simulink model "Force_control_impedance"  (R2020b)
settings: Solver=VariableStepAuto  StartTime=0.0  StopTime=.1  RelTol=1e-3
settings Model: Creator=Jae  LastModifiedBy=Jae

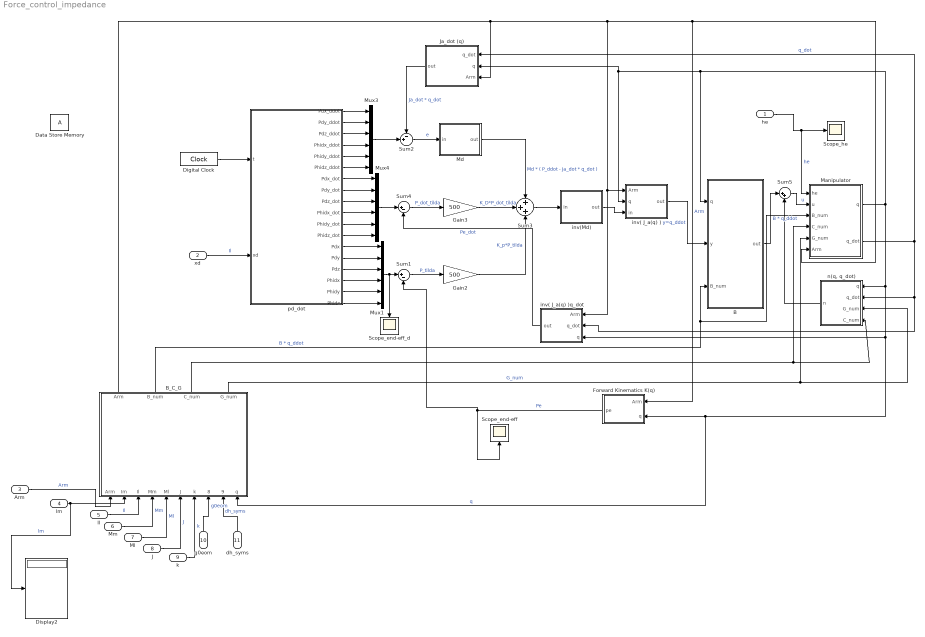
== system Force_control_impedance ==
  he : Inport  PortDimensions=6  SampleTime=0.01
  xd : Inport  Port=2  PortDimensions=6  SampleTime=0.01
  Arm : Inport  Port=3  PortDimensions=6  SampleTime=0.01
  lm : Inport  Port=4  PortDimensions=6  SampleTime=0.01
  Il : Inport  Port=5  PortDimensions=6  SampleTime=0.01
  Mm : Inport  Port=6  PortDimensions=6  SampleTime=0.01
  Ml : Inport  Port=7  PortDimensions=6  SampleTime=0.01
  J : Inport  Port=8  PortDimensions=6  SampleTime=0.01
  k : Inport  Port=9  PortDimensions=6  SampleTime=0.01
  g0eom : Inport  Port=10  PortDimensions=6  SampleTime=0.01
  dh_syms : Inport  Port=11  PortDimensions=6  SampleTime=0.01
  B : MATLAB Function  TreatAsAtomicUnit=on
  B_C_G : MATLAB Function  TreatAsAtomicUnit=on
  Data Store Memory : DataStoreMemory  ReadBeforeWriteMsg=warning  WriteAfterWriteMsg=warning  WriteAfterReadMsg=warning  ShowAdditionalParam=off
  Digital Clock : DigitalClock  SampleTime=0.01
  Display2 : Display
  Forward Kinematics K(q) : MATLAB Function  TreatAsAtomicUnit=on
  Gain2 : Gain  Gain=500
  Gain3 : Gain  Gain=500
  Ja_dot (q) : MATLAB Function  TreatAsAtomicUnit=on
  Manipulator : Subsystem
  Md : MATLAB Function  TreatAsAtomicUnit=on
  Mux1 : Mux  Inputs=6
  Mux3 : Mux  Inputs=6
  Mux4 : Mux  Inputs=6
  Scope_end-eff : Scope
  Scope_end-eff_d : Scope
  Scope_he : Scope
  Sum1 : Sum  Inputs=|+-
  Sum2 : Sum  Inputs=-+|
  Sum3 : Sum  Inputs=+++
  Sum4 : Sum  Inputs=|+-
  Sum5 : Sum  Inputs=|++
  inv( J_a(q) ) : MATLAB Function  TreatAsAtomicUnit=on
  inv( J_a(q) )q_dot : MATLAB Function  TreatAsAtomicUnit=on
  inv(Md) : MATLAB Function  TreatAsAtomicUnit=on
  "n(q, q_dot)" : Subsystem
  pd_dot : MATLAB Function  TreatAsAtomicUnit=on
  wires:
  Digital Clock/1 -> pd_dot/1(t)
  inv( J_a(q) )/1(out) -> B/2(y)  "y=q_ddot"
  pd_dot/13(Pdx) -> Mux1/1
  pd_dot/14(Pdy) -> Mux1/2
  pd_dot/15(Pdz) -> Mux1/3
  pd_dot/16(Phidx) -> Mux1/4
  pd_dot/17(Phidy) -> Mux1/5
  pd_dot/18(Phidz) -> Mux1/6
  pd_dot/1(Pdx_ddot) -> Mux3/1
  pd_dot/2(Pdy_ddot) -> Mux3/2
  pd_dot/3(Pdz_ddot) -> Mux3/3
  pd_dot/4(Phidx_ddot) -> Mux3/4
  pd_dot/5(Phidy_ddot) -> Mux3/5
  pd_dot/6(Phidz_ddot) -> Mux3/6
  pd_dot/7(Pdx_dot) -> Mux4/1
  pd_dot/8(Pdy_dot) -> Mux4/2
  pd_dot/9(Pdz_dot) -> Mux4/3
  pd_dot/10(Phidx_dot) -> Mux4/4
  pd_dot/11(Phidy_dot) -> Mux4/5
  pd_dot/12(Phidz_dot) -> Mux4/6
  Gain3/1 -> Sum3/2  "K_D*P_dot_tilda"
  Mux3/1 -> Sum2/2
  Sum2/1 -> Md/1(in)  "e"
  Md/1(out) -> Sum3/1  "Md * ( P_ddot - Ja_dot * q_dot )"
  Mux4/1 -> Sum4/1
  Sum4/1 -> Gain3/1  "P_dot_tilda"
  Mux1/1 -> Scope_end-eff_d/1, Sum1/1
  Sum1/1 -> Gain2/1  "P_tilda"
  Sum3/1 -> inv(Md)/1(in)
  Gain2/1 -> Sum3/3  "K_p*P_tilda"
  inv(Md)/1(out) -> inv( J_a(q) )/3(in)
  Ja_dot (q)/1(out) -> Sum2/1  "Ja_dot * q_dot"
  Forward Kinematics K(q)/1(pe) -> Sum1/2, Scope_end-eff/1  "Pe"
  inv( J_a(q) )q_dot/1(out) -> Sum4/2  "Pe_dot"
  B/1(out) -> Sum5/1  "B * q_ddot"
  "n(q, q_dot)"/1(n) -> Sum5/2
  Manipulator/1(q) -> B/1(q), inv( J_a(q) )/2(q), Ja_dot (q)/2(q), Forward Kinematics K(q)/2(q), B_C_G/10(q), inv( J_a(q) )q_dot/3(q), "n(q, q_dot)"/1(q)  "q"
  Manipulator/2(q_dot) -> Ja_dot (q)/1(q_dot), inv( J_a(q) )q_dot/2(q_dot), "n(q, q_dot)"/2(q_dot)  "q_dot"
  Sum5/1 -> Manipulator/2(u)  "u"
  he/1 -> Scope_he/1, Manipulator/1(he)  "he"
  Arm/1 -> B_C_G/1("Arm ")  "Arm"
  lm/1 -> Display2/1, B_C_G/2(Im)  "lm"
  Il/1 -> B_C_G/3(Il)  "Il"
  Mm/1 -> B_C_G/4(Mm)  "Mm"
  Ml/1 -> B_C_G/5(Ml)  "Ml"
  J/1 -> B_C_G/6(J)  "J"
  k/1 -> B_C_G/7(k)  "k"
  g0eom/1 -> B_C_G/8(g0eom)  "g0eom"
  dh_syms/1 -> B_C_G/9(dh_syms)  "dh_syms"
  B_C_G/2(B_num) -> B/3(B_num), Manipulator/3(B_num)  "B * q_ddot"
  B_C_G/1(Arm) -> Ja_dot (q)/3(Arm), Forward Kinematics K(q)/1(Arm), Manipulator/6(Arm), inv( J_a(q) )q_dot/1(Arm), inv( J_a(q) )/1(Arm)  "Arm"
  B_C_G/4(G_num) -> Manipulator/5(G_num), "n(q, q_dot)"/3(G_num)  "G_num"
  B_C_G/3(C_num) -> Manipulator/4(C_num), "n(q, q_dot)"/4(C_num)
  xd/1 -> pd_dot/2(xd)  "Il"

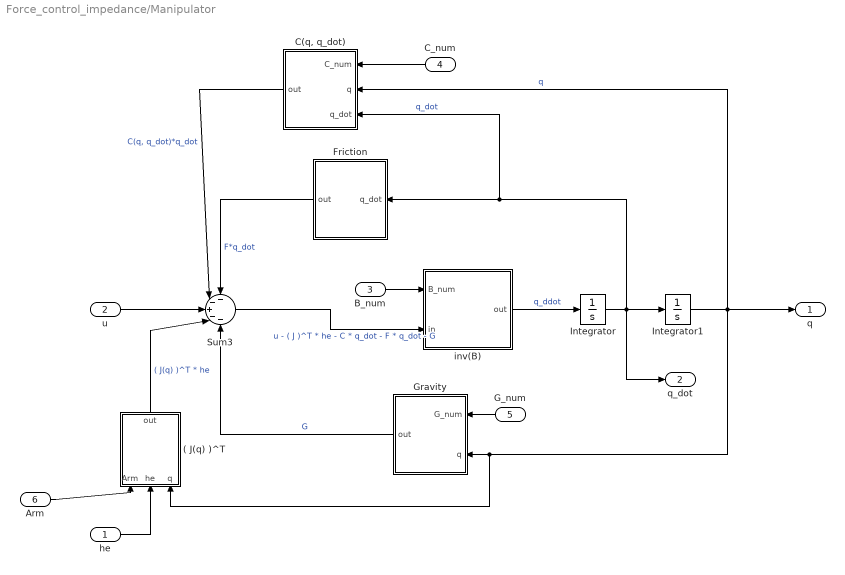
== system Force_control_impedance/Manipulator ==
  he : Inport
  u : Inport  Port=2
  B_num : Inport  Port=3
  C_num : Inport  Port=4
  G_num : Inport  Port=5
  Arm : Inport  Port=6
  ( J(q) )^T : MATLAB Function  TreatAsAtomicUnit=on
  "C(q, q_dot)" : MATLAB Function  TreatAsAtomicUnit=on
  Friction : MATLAB Function  TreatAsAtomicUnit=on
  Gravity : MATLAB Function  TreatAsAtomicUnit=on
  Integrator : Integrator  InitialCondition=[0 0 0 0 0 0]'  ZeroCross=off
  Integrator1 : Integrator  InitialCondition=[0 0 0 0 0 0]'  ZeroCross=off
  Sum3 : Sum  Inputs=--+--
  inv(B) : MATLAB Function  TreatAsAtomicUnit=on
  q : Outport
  q_dot : Outport  Port=2
  wires:
  u/1 -> Sum3/3
  ( J(q) )^T/1(out) -> Sum3/4  "( J(q) )^T * he"
  "C(q, q_dot)"/1(out) -> Sum3/2  "C(q, q_dot)*q_dot"
  Friction/1(out) -> Sum3/1  "F*q_dot"
  inv(B)/1(out) -> Integrator/1  "q_ddot"
  Integrator/1 -> Integrator1/1, q_dot/1, Friction/1(q_dot), "C(q, q_dot)"/3(q_dot)  "q_dot"
  Integrator1/1 -> Gravity/2(q), ( J(q) )^T/3(q), "C(q, q_dot)"/2(q), q/1  "q"
  Sum3/1 -> inv(B)/2(in)  "u - ( J )^T * he - C * q_dot - F * q_dot - G"
  Gravity/1(out) -> Sum3/5  "G"
  he/1 -> ( J(q) )^T/2(he)
  B_num/1 -> inv(B)/1(B_num)
  C_num/1 -> "C(q, q_dot)"/1(C_num)
  G_num/1 -> Gravity/1(G_num)
  Arm/1 -> ( J(q) )^T/1(Arm)

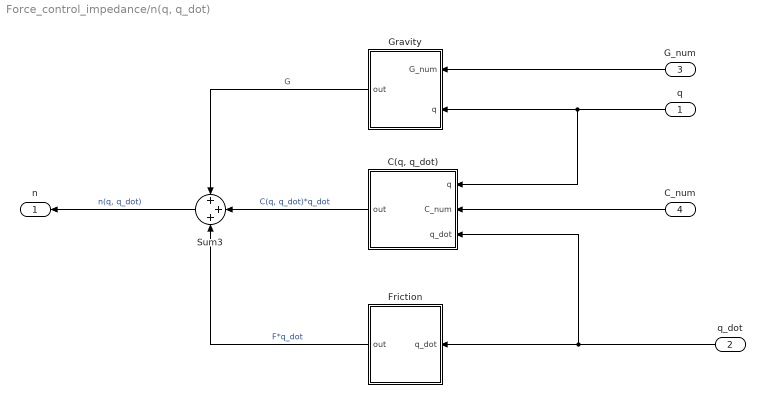
== system Force_control_impedance/n(q, q_dot) ==
  q : Inport
  q_dot : Inport  Port=2
  G_num : Inport  Port=3
  C_num : Inport  Port=4
  "C(q, q_dot)" : MATLAB Function  TreatAsAtomicUnit=on
  Friction : MATLAB Function  TreatAsAtomicUnit=on
  Gravity : MATLAB Function  TreatAsAtomicUnit=on
  Sum3 : Sum  Inputs=+++
  n : Outport
  wires:
  Sum3/1 -> n/1  "n(q, q_dot)"
  Gravity/1(out) -> Sum3/1  "G"
  "C(q, q_dot)"/1(out) -> Sum3/2  "C(q, q_dot)*q_dot"
  Friction/1(out) -> Sum3/3  "F*q_dot"
  q/1 -> "C(q, q_dot)"/1(q), Gravity/2(q)
  q_dot/1 -> "C(q, q_dot)"/3(q_dot), Friction/1(q_dot)
  G_num/1 -> Gravity/1(G_num)
  C_num/1 -> "C(q, q_dot)"/2(C_num)

== matlab function Force_control_impedance/inv( J_a(q) )q_dot ==
  data: Arm input; q_dot input; out output; q input
function out = Ja(Arm, q_dot, q)
%{
Inputs:
in: q_dot, q
    nx1    nx1             
Output: Ja*q_dot;
        6xn*nx1 = 6x1
%}
Ja = jacob0(Arm, q', 'rpy'); % 6xn

out = Ja*q_dot;
end

== matlab function Force_control_impedance/n(q, q_dot)/C(q, q_dot) ==
  data: q input; C_num input; q_dot input; out output
function out = C(q, C_num, q_dot)
% need to calculate C

out=C_num*q_dot;
end

== matlab function Force_control_impedance/n(q, q_dot)/Gravity ==
  data: G_num input; q input; out output
function out = G(G_num, q)
out=G_num;
end

== matlab function Force_control_impedance/n(q, q_dot)/Friction ==
  data: q_dot input; out output
function out = F(q_dot)
%{
Inputs:
in: q_dot
    nx1                
Output: F * q_dot;
        nxn*nx1 = nx1
%}
%NOTE: Assumed Arm,Im,Il,Mm,Ml,J,k,g0eom,dh_syms are global variables
%[B,C,G] = EOMFinder(Arm,Im,Il,Mm,Ml,J,k,g0eom,dh_syms);
%function Fv = Friction(FB, Fpos, Fneg, dq, n)
%F is friction is  NxN
%n=size(FB,1);
%assert (n <= 20);
%create vector of friction coefficients
n=length(q0)
FB=0; Fpos=0; Fneg=0; 
F_vector=zeros(n,1);

for i=1:n
    if dq(i)>0
        F_vector(i)= FB*dq(i)+Fpos;
    elseif dq(i)<0 % 
        F_vector(i)= FB*dq(i)+Fneg;
    else %         -        +
        F_vector(i)=0;
    end
end

%convert F_vector to diagonal matrix
F_diag=diag(F_vector);

%out is Nx1
out=zeros(n,1);
out=F_diag;

end

== matlab function Force_control_impedance/B_C_G ==
  data: Arm output; B_num output; Arm input; Im input; Il input; Mm input; Ml input; J input; k input; g0eom input; dh_syms input; q input; C_num output; G_num output
function [Arm, B_num, C_num, G_num] = B_C_G(Arm,Im,Il,Mm,Ml,J,k,g0eom,dh_syms, q)
%{
Inputs:
in: q,     y (q_ddot)
    nx1    nx1             
Output: B*y;
        nxn*nx1 = nx1
%}
%NOTE: Assumed Arm,Im,Il,Mm,Ml,J,k,g0eom,dh_syms are global variables
[B,C,G] = EOMFinder(Arm,Im,Il,Mm,Ml,J,k,g0eom,dh_syms);
Arm;
B_num=BFinder(B,q');
C_num=CFinder(C,q');
G_num=GFinder(G,q');


end

== matlab function Force_control_impedance/Manipulator/( J(q) )^T ==
  data: Arm input; out output; he input; q input
function out = J_T(Arm, he, q)
%{
Inputs:
in: q,     y (q_ddot)
    nx1    nx1             
Output: B*y;
        nxn*nx1 = nx1
%}
% need to define he 6x1 he
if isempty(q)==1
    n=length(q);
    q=ones(1,n);
end

disp(he)
J=Arm.jacob0(q'); 
% 6xn 
out = zeros(6,1);
out = J'*he;
  %  nx6*6x1 = nx1
end

== matlab function Force_control_impedance/Manipulator/C(q, q_dot) ==
  data: C_num input; q input; q_dot input; out output
function out = C(C_num, q,q_dot)
%{
Inputs:
in: q,     q_dot
    nx1    nx1             
Output: C_num*q_dot;
        nxn  *nx1 = nx1
%}
%NOTE: Assumed Arm,Im,Il,Mm,Ml,J,k,g0eom,dh_syms are global variables
% [B,C,G] = EOMFinder(Arm,Im,Il,Mm,Ml,J,k,g0eom,dh_syms);
% C_num=CFinder(C,q');
out=C_num*q_dot;
end

== matlab function Force_control_impedance/Manipulator/Friction ==
  data: q_dot input; out output
function out = F(q_dot)
%{
Inputs:
in: q_dot
    nx1                
Output: F * q_dot;
        nxn*nx1 = nx1
%}
%NOTE: Assumed Arm,Im,Il,Mm,Ml,J,k,g0eom,dh_syms are global variables
%[B,C,G] = EOMFinder(Arm,Im,Il,Mm,Ml,J,k,g0eom,dh_syms);
%function Fv = Friction(FB, Fpos, Fneg, dq, n)
%F is friction is  NxN
%n=size(FB,1);
%assert (n <= 20);
%create vector of friction coefficients
n=length(q0)
FB=0; Fpos=0; Fneg=0; 
F_vector=zeros(n,1);

for i=1:n
    if dq(i)>0
        F_vector(i)= FB*dq(i)+Fpos;
    elseif dq(i)<0 % 
        F_vector(i)= FB*dq(i)+Fneg;
    else %         -        +
        F_vector(i)=0;
    end
end

%convert F_vector to diagonal matrix
F_diag=diag(F_vector);

%out is Nx1
out=zeros(n,1);
out=F_diag;

end

== matlab function Force_control_impedance/Manipulator/Gravity ==
  data: G_num input; q input; out output
function out = G(G_num,q)
% need to calculate G
%{
Inputs:
in: in
    nx1              
Output: pinv(B)*in;
        nxn*nx1 = nx1
%}
%NOTE: Assumed Arm,Im,Il,Mm,Ml,J,k,g0eom,dh_syms are global variables
% [B,C,G] = EOMFinder(Arm,Im,Il,Mm,Ml,J,k,g0eom,dh_syms);
% G_num=GFinder(G,q');
out=G_num;
end

== matlab function Force_control_impedance/B ==
  data: q input; y input; out output; B_num input
function out = B(q, y, B_num)
%{
Inputs:
in: q,     y (q_ddot)
    nx1    nx1             
Output: B*y;
        nxn*nx1 = nx1
%}
%NOTE: Assumed Arm,Im,Il,Mm,Ml,J,k,g0eom,dh_syms are global variables
%[B,C,G] = EOMFinder(Arm,Im,Il,Mm,Ml,J,k,g0eom,dh_syms);
%B_num=BFinder(B,q');
out=B_num*y;
end

== matlab function Force_control_impedance/Md ==
  data: in input; out output
% Multiply by Md
function out = Md(in)
%{
Inputs:
in: Ja_dot * q_dot
    6xn    * nx1

Output: Md*in
       6x6*6x1=6x1
%}
input=[2 2 2 2 2 2];
Md = diag(input);
                        
out = Md * in; % 6x1
end

== matlab function Force_control_impedance/inv(Md) ==
  data: in input; out output
% Multiply by inv(Md)
function out = invMd(in)
%{
Inputs:
in: Md * ( P_ddot - Ja_dot * q_dot ) + K_D*P_dot_tilda + K_p*P_tilda
    6x6   * (6x1  - 6x6    * 6x1 )   + 6x1             + 6x1 
    Md * (x_dd    - Ja_dot * q_dot ) + K_D*x_dot_tilda + K_p*x_tilda                        
Output: inv(Md)*in
       6x6*6x1=6x1
%}
input=[2 2 2 2 2 2];

Md = diag(input);
% psuedo-inverse just in case when Md is not 6x6 mat
out = pinv(Md)*in;
end

== matlab function Force_control_impedance/Ja_dot (q) ==
  data: q_dot input; out output; q input; Arm input
function out = Ja_dot(q_dot, q, Arm)
%{
Inputs:
q_dot: nx1
q: nx1 

Output: Analytical Jacobian
Ja_dot = jacob_dot(Arm, q', q_dot');
- Takes 1xn form of each q and q_dot
%}
Ja_dot = jacob_dot(Arm, q', q_dot');

out = Ja_dot*q_dot;
end

== matlab function Force_control_impedance/pd_dot ==
  data: Pdx_ddot output; Pdy_ddot output; Pdz_ddot output; Phidx_ddot output; Phidy_ddot output; Phidz_ddot output; Pdx_dot output; Pdy_dot output; Pdz_dot output; Phidx_dot output; Phidy_dot output; Phidz_dot output; t input; Pdx output; Pdy output; Pdz output; Phidx output; Phidy output; Phidz output; xd input
function [Pdx_ddot,Pdy_ddot,Pdz_ddot,Phidx_ddot,Phidy_ddot,Phidz_ddot,Pdx_dot,Pdy_dot,Pdz_dot,Phidx_dot,Phidy_dot,Phidz_dot,Pdx,Pdy,Pdz,Phidx,Phidy,Phidz] = pos_vel_acc(t, xd)
% Pd
% syms t
xd(1)
Pdx=xd(1);
Pdy=xd(2);
Pdz=xd(3);
Phidx=xd(4);
Phidy=xd(5);
Phidz=xd(6);
% Pd_dot
Pdx_dot=0;
Pdy_dot=0;
Pdz_dot=0;
Phidx_dot=0;
Phidy_dot=0;
Phidz_dot=0;
% Pd_ddot
Pdx_ddot=0;
Pdy_ddot=0;
Pdz_ddot=0;
Phidx_ddot=0;
Phidy_ddot=0;
Phidz_ddot=0;

% % Pd_dot
% Pdx_dot=diff(Pdx,t);
% Pdy_dot=diff(Pdy,t);
% Pdz_dot=diff(Pdz,t);
% Phidx_dot=diff(Phidx,t);
% Phidy_dot=diff(Phidy,t);
% Phidz_dot=diff(Phidz,t);
% % Pd_ddot
% Pdx_ddot=diff(Pdx_dot,t);
% Pdy_ddot=diff(Pdy_dot,t);
% Pdz_ddot=diff(Pdz_dot,t);
% Phidx_ddot=diff(Phidx_dot,t);
% Phidy_ddot=diff(Phidy_dot,t);
% Phidz_ddot=diff(Phidz_dot,t);
end

== matlab function Force_control_impedance/Manipulator/inv(B) ==
  data: B_num input; in input; out output
function out = invB(B_num, in)
% need to calculate B
%{
Inputs:
in: in
    nx1              
Output: pinv(B)*in;
        nxn*nx1 = nx1
%}
if isempty(in)==1
    n=length(in);
    q=ones(1,n);
end

%NOTE: Assumed Arm,Im,Il,Mm,Ml,J,k,g0eom,dh_syms are global variables
% [B,C,G] = EOMFinder(Arm,Im,Il,Mm,Ml,J,k,g0eom,dh_syms);
% B_num=BFinder(B,q);
out=pinv(B_num)*in;
%      nxn * nx1
end

== matlab function Force_control_impedance/Forward Kinematics K(q) ==
  data: Arm input; q input; pe output
function pe = f_kin(Arm, q)
%{
Inputs:
in: q
    nx1             
Output: 4x4
%}
if isempty(q)==1
    q = [-2.8210 -2.9561 6.5625]';
end
Arm
% q=[1 1 1]'
q
T=Arm.fkine(q);
% roll pitch yaw
rpy=tr2rpy(T);
p=transl(T);
%xe: 6 x 1 vector of actual 6-DOF arm position
pe=zeros(6, 1);
pe=[p(1); p(2); p(3); rpy(1); rpy(2); rpy(3)];
% pe=eval(pe);

end

== matlab function Force_control_impedance/inv( J_a(q) ) ==
  data: Arm input; q input; in input; out output
function out = invJa(Arm, q, in)
%{
Inputs:
in: q,     in
    nx1    6x1             
Output: pinv(Ja)*in;
        6xn*nx1 = 6x1
%}
Ja = jacob0(Arm, q', 'rpy'); % 6xn

out = pinv(Ja)*in;
%     nx6     *6x1   = nx1
end
